simulink model "M4_P1"  (R2023a)
settings: Solver=VariableStepAuto  StartTime=0.0  StopTime=10  RelTol=1e-3
values from neighbouring files (symbols this model uses):
  f_eff = 0.001 + (0.001 * NRP)    [M4_Script.m]
  inputx = pos_ref_values_tugas(i,1)    [M4_Script.m]
  inputy = pos_ref_values_tugas(i,2)    [M4_Script.m]
  J_eff = 0.00004 + (0.00001 * NRP)    [M4_Script.m]
  Kb = 0.02 + (0.001 * NRP)    [M4_Script.m]
  Ktn = 0.026 + (0.001 * NRP)    [M4_Script.m]
  L = 0.062    [M4_Script.m]
  l1 = 33    [M4_Script.m]
  l2 = 25    [M4_Script.m]
  R = 2.5    [M4_Script.m]
settings Model: Creator=azzam  LastModifiedBy=azzam
settings DebuggingCC: AlgebraicLoopMsg=none

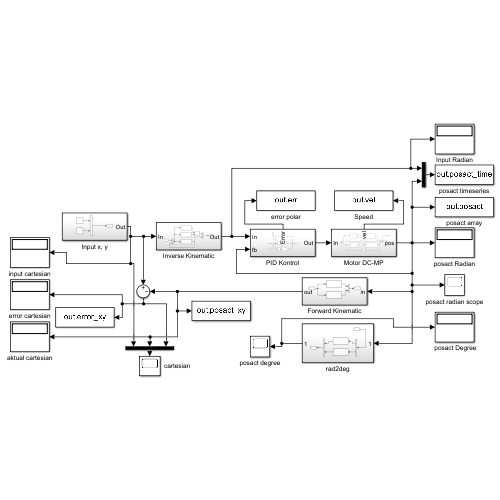
[thumbnail: Simulink's stored preview of the top-level diagram]
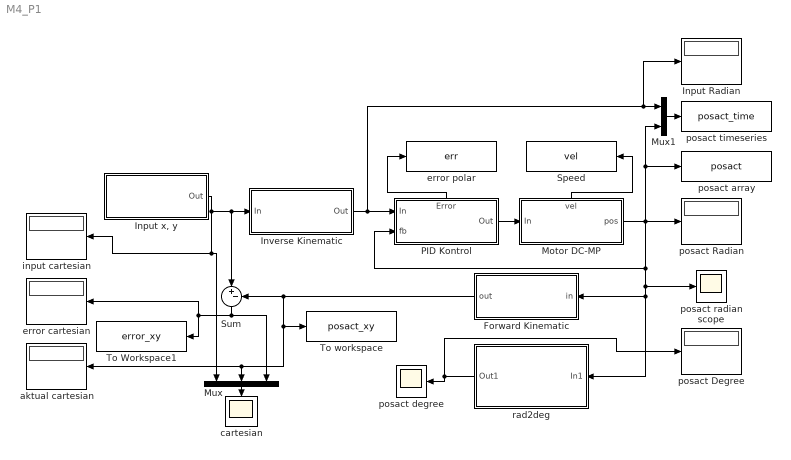
== system M4_P1 ==
  " posact Degree" : Display
  Forward Kinematic : Subsystem
  Input Radian : Display
  "Input x, y" : Subsystem
  Inverse Kinematic : Subsystem
  Motor DC-MP : Subsystem
      settings: PortSchema="{\"entries\":[{\"content\":{\"sides\":[{\"content\":{\"connectorIds\":[\"In1\"]},\"type\":\"ConnectorPlacement.EquallySpacedRectSide\",\"uuid\":\"ac7a8215-a36d-4697-93b9-89f5dd1873e2\"},{\"content\":{\"connectorIds\":[\"Out1\"],\"side\":\"RIGHT\"},\"type\":\"ConnectorPlacement.EquallySpacedRectSide\",\"uuid\":\"e6865d54-49ab-4755-a29e-3873af484436\"},{\"content\":{\"connectorIds\":[\"Out2\"],\"side\":\"TOP\"},\"type\":\"ConnectorPlacement.EquallySpacedRectSide\",\"uuid\":\"422b713d-6d9a-4f85-a64b-19f888d04706\"}]},\"type\":\"ConnectorPlacement.EquallySpacedConnector\",\"uuid\":\"c603a5fe-1fe0-45df-906e-a54f41e56c56\"}],\"packageUris\":[\"http://schema.mathworks.com/mf0/Connector/R2020b\"],\"version\":\"1.0\"}"
  Mux : Mux  Inputs=3
  Mux1 : Mux  Inputs=2
  PID Kontrol : Subsystem
      settings: PortSchema="{\"entries\":[{\"content\":{\"sides\":[{\"content\":{\"connectorIds\":[\"In1\",\"In2\"]},\"type\":\"ConnectorPlacement.EquallySpacedRectSide\",\"uuid\":\"555cc180-eba4-4e10-983a-f071b59ba1a6\"},{\"content\":{\"connectorIds\":[\"Out1\"],\"side\":\"RIGHT\"},\"type\":\"ConnectorPlacement.EquallySpacedRectSide\",\"uuid\":\"484a5ffc-25a4-4c1d-993c-003812c9027a\"},{\"content\":{\"connectorIds\":[\"Out2\"],\"side\":\"TOP\"},\"type\":\"ConnectorPlacement.EquallySpacedRectSide\",\"uuid\":\"87f69f45-c544-4588-a580-9a9c1b01860f\"}]},\"type\":\"ConnectorPlacement.EquallySpacedConnector\",\"uuid\":\"8fe3331b-1a8a-473f-ba9e-387282cc206b\"}],\"packageUris\":[\"http://schema.mathworks.com/mf0/Connector/R2020b\"],\"version\":\"1.0\"}"
  Speed : ToWorkspace  VariableName=vel  SaveFormat=Timeseries  SampleTime=-1
      settings: Save2DSignal=2-D array (concatenate along first dimension)
  Sum : Sum  Inputs=|+-
  To Workspace1 : ToWorkspace  VariableName=error_xy  SampleTime=-1
      settings: Save2DSignal=2-D array (concatenate along first dimension)
  To workspace : ToWorkspace  VariableName=posact_xy  SampleTime=-1
      settings: Save2DSignal=2-D array (concatenate along first dimension)
  aktual cartesian : Display
  cartesian : Scope
  error cartesian : Display
  error polar : ToWorkspace  VariableName=err  SaveFormat=Timeseries  SampleTime=-1
      settings: Save2DSignal=2-D array (concatenate along first dimension)
  input cartesian : Display
  posact Radian : Display
  posact array : ToWorkspace  VariableName=posact  SampleTime=-1
      settings: Save2DSignal=2-D array (concatenate along first dimension)
  posact degree : Scope
  posact radian scope : Scope
  posact timeseries : ToWorkspace  VariableName=posact_time  SaveFormat=Timeseries  SampleTime=-1
      settings: Save2DSignal=2-D array (concatenate along first dimension)
  rad2deg : Subsystem
  wires:
  Inverse Kinematic/1(Out) -> Mux1/1, Input Radian/1, PID Kontrol/1(In)
  PID Kontrol/1(Out) -> Motor DC-MP/1(In)
  Motor DC-MP/1(pos) -> Mux1/2, posact array/1, rad2deg/1(In1), Forward Kinematic/1(in), posact radian scope/1, PID Kontrol/2(fb), posact Radian/1
  Sum/1 -> error cartesian/1, To Workspace1/1, Mux/3
  Mux/1 -> cartesian/1
  Forward Kinematic/1(out) -> Sum/2, aktual cartesian/1, Mux/2, To workspace/1
  "Input x, y"/1(Out) -> Inverse Kinematic/1(In), Sum/1, Mux/1, input cartesian/1
  Motor DC-MP/2(vel) -> Speed/1
  Mux1/1 -> posact timeseries/1
  rad2deg/1(Out1) -> posact degree/1, " posact Degree"/1
  PID Kontrol/2(Error) -> error polar/1

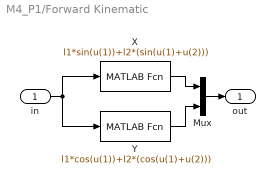
== system M4_P1/Forward Kinematic ==
  in : Inport
  Mux : Mux  Inputs=2
  X : MATLABFcn  MATLABFcn=l1*sin(u(1))+l2*(sin(u(1)+u(2)))
  Y : MATLABFcn  MATLABFcn=l1*cos(u(1))+l2*(cos(u(1)+u(2)))
  out : Outport
  wires:
  Mux/1 -> out/1
  X/1 -> Mux/1
  Y/1 -> Mux/2
  in/1 -> Y/1, X/1

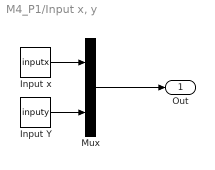
== system M4_P1/Input x, y ==
  Input Y : Constant  Value=inputy
  Input x : Constant  Value=inputx
  Mux : Mux  Inputs=2
  Out : Outport
  wires:
  Input x/1 -> Mux/1
  Input Y/1 -> Mux/2
  Mux/1 -> Out/1

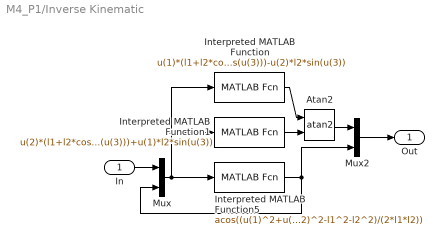
== system M4_P1/Inverse Kinematic ==
  In : Inport
  Atan2 : Trigonometry  Operator=atan2
  Interpreted MATLAB Function : MATLABFcn  MATLABFcn=u(1)*(l1+l2*cos(u(3)))-u(2)*l2*sin(u(3))
  Interpreted MATLAB Function1 : MATLABFcn  MATLABFcn=u(2)*(l1+l2*cos(u(3)))+u(1)*l2*sin(u(3))
  Interpreted MATLAB Function5 : MATLABFcn  MATLABFcn=acos((u(1)^2+u(2)^2-l1^2-l2^2)/(2*l1*l2))
  Mux : Mux  Inputs=2
  Mux2 : Mux  Inputs=2
  Out : Outport
  wires:
  In/1 -> Mux/1
  Mux2/1 -> Out/1
  Interpreted MATLAB Function5/1 -> Mux/2, Mux2/2
  Atan2/1 -> Mux2/1
  Interpreted MATLAB Function1/1 -> Atan2/2
  Mux/1 -> Interpreted MATLAB Function5/1, Interpreted MATLAB Function/1, Interpreted MATLAB Function1/1
  Interpreted MATLAB Function/1 -> Atan2/1

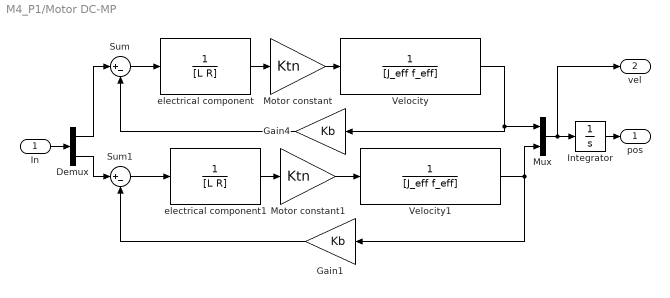
== system M4_P1/Motor DC-MP ==
  In : Inport
  Demux : Demux  Outputs=2
  Gain1 : Gain  Gain=Kb
  Gain4 : Gain  Gain=Kb
  Integrator : Integrator
  Motor constant : Gain  Gain=Ktn
  Motor constant1 : Gain  Gain=Ktn
  Mux : Mux  Inputs=2
  Sum : Sum  Inputs=|+-
  Sum1 : Sum  Inputs=|+-
  Velocity : TransferFcn  Denominator=[J_eff f_eff]
  Velocity1 : TransferFcn  Denominator=[J_eff f_eff]
  electrical component : TransferFcn  Denominator=[L R]
  electrical component1 : TransferFcn  Denominator=[L R]
  pos : Outport
  vel : Outport  Port=2
  wires:
  In/1 -> Demux/1
  Integrator/1 -> pos/1
  Mux/1 -> vel/1, Integrator/1
  Demux/1 -> Sum/1
  Demux/2 -> Sum1/1
  Velocity/1 -> Mux/1, Gain4/1
  electrical component/1 -> Motor constant/1
  Motor constant/1 -> Velocity/1
  Sum/1 -> electrical component/1
  Gain4/1 -> Sum/2
  Gain1/1 -> Sum1/2
  Velocity1/1 -> Gain1/1, Mux/2
  Sum1/1 -> electrical component1/1
  Motor constant1/1 -> Velocity1/1
  electrical component1/1 -> Motor constant1/1

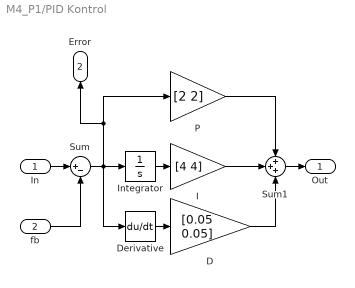
== system M4_P1/PID Kontrol ==
  In : Inport
  fb : Inport  Port=2
  D : Gain  Gain=[0.05 0.05]
  Derivative : Derivative
  I : Gain  Gain=[4 4]
  Integrator : Integrator
  P : Gain  Gain=[2 2]
  Sum : Sum  Inputs=|+-
  Sum1 : Sum  Inputs=+++
  Out : Outport
  Error : Outport  Port=2
  wires:
  In/1 -> Sum/1
  fb/1 -> Sum/2
  Sum1/1 -> Out/1
  P/1 -> Sum1/1
  Sum/1 -> Derivative/1, Integrator/1, Error/1, P/1
  D/1 -> Sum1/3
  I/1 -> Sum1/2
  Integrator/1 -> I/1
  Derivative/1 -> D/1

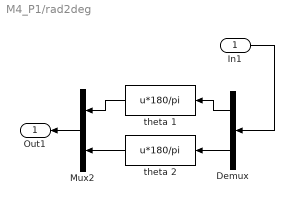
== system M4_P1/rad2deg ==
  In1 : Inport
  Demux : Demux  Outputs=2
  Mux2 : Mux  Inputs=2
  theta 1 : MATLABFcn  MATLABFcn=u*180/pi
  theta 2 : MATLABFcn  MATLABFcn=u*180/pi
  Out1 : Outport
  wires:
  Demux/1 -> theta 1/1
  theta 1/1 -> Mux2/1
  In1/1 -> Demux/1
  theta 2/1 -> Mux2/2
  Demux/2 -> theta 2/1
  Mux2/1 -> Out1/1
